simulink model "powerline_cycle_waterfall_milestone_06"  (R2026a)
settings: Solver=VariableStepAuto  StopTime=59/60
model workspace (MAT data in the model file):
  noiseGain = 1
  sparkGain = 1
undefined symbols (not defined in the file): fs
libraries: dspsrcs4 x3
settings Model: PacingRate=0.100000  Creator=docto  LastModifiedBy=docto

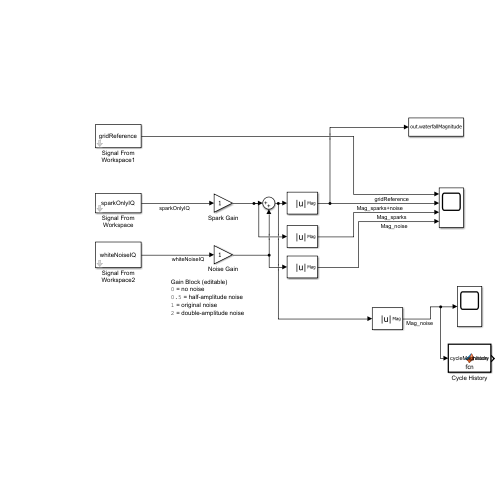
[thumbnail: Simulink's stored preview of the top-level diagram]
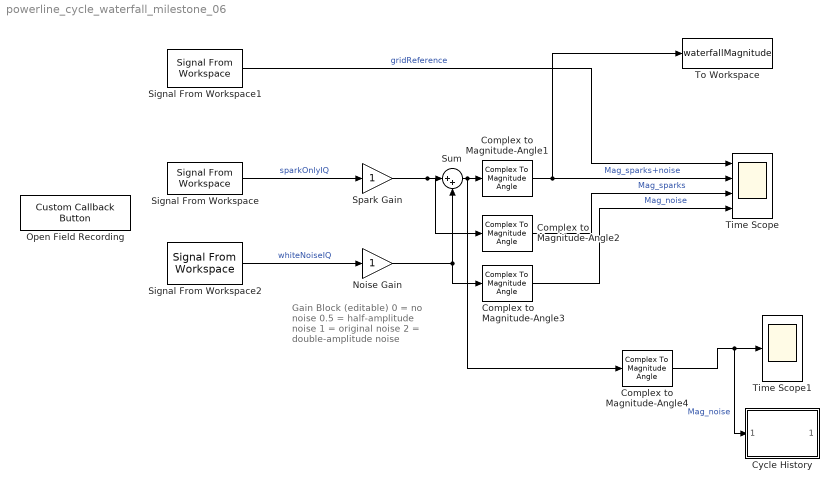
== system powerline_cycle_waterfall_milestone_06 ==
  note: Gain Block (editable)
      | 0 = no noise
      | 0.5 = half-amplitude noise
      | 1 = original noise
      | 2 = double-amplitude noise
  Complex to Magnitude-Angle{1..4} (4 alike) : ComplexToMagnitudeAngle  Output=Magnitude
  Cycle History : MATLAB Function  TreatAsAtomicUnit=on
  Noise Gain : Gain
  Open Field Recording : CustomCallbackButton  Configuration="{\"components\":[{\"name\":\"BackgroundImageComponent\",\"settings\":{\"image\":{\"size\":[0,0],\"src\":\"default\",\"srcOrientation\":\"Right\"},\"position\":[0,0,1,1]}},{\"name\":\"ButtonStateComponent\",\"settings\":{\"buttonType\":\"momentary\",\"clickFcn\":\"openFieldEventWaterfall;\",\"onValue\":1,\"position\":[0,0,1,1],\"pressDelay\":\"500\",\"pressFcn\":\"\",\"repeatInterval\":\"0\",\"states\":[{\"horizontalAlignment\":\"center\",\"image\":{\"position\":[0,0,1,1],\"size\":[1,1],\"src\":\"default\",\"srcOrientation\":\"Right\"},\"label\":{\"color\":[0.01176470588,0.01176470588,0.01176470588,1],\"icon\":{\"size\":[0,0],\"src\":\"default\",\"srcOrientation\":\"Right\"},\"iconOffset\":0,\"iconPlacement\":\"left\",\"opacity\":1,\"show\":true,\"text\":{\"content\":\"Open Field Recording\",\"font\":\"Helvetica\"}},\"labelOffset\":[0,0],\"verticalAlignment\":\"middle\"},{\"horizontalAlignment\":\"center\",\"image\":{\"position\":[0,0,1,1],\"size\":[1,1],\"src\":\"default\",\"srcOrientation\":\"Right\"},\"label\":{\"color\":[0.01176470588,0.01176470588,0.01176470588,1],\"icon\":{\"size\":[0,0],\"src\":\"default\",\"srcOrientation\":\"Right\"},\"iconOffset\":0,\"iconPlacement\":\"left\",\"opacity\":1,\"show\":true,\"text\":{\"content\":\"Open Field Recording\",\"font\":\"Helvetica\"}},\"labelOffset\":[0,0],\"verticalAlignment\":\"middle\"},{\"horizontalAlignment\":\"center\",\"image\":{\"position\":[0,0,1,1],\"size\":[1,1],\"src\":\"default\",\"srcOrientation\":\"Right\"},\"label\":{\"color\":[0.01176470588,0.01176470588,0.01176470588,1],\"icon\":{\"size\":[0,0],\"src\":\"default\",\"srcOrientation\":\"Right\"},\"iconOffset\":0,\"iconPlacement\":\"left\",\"opacity\":1,\"show\":true,\"text\":{\"content\":\"Open Field Recording\",\"font\":\"Helvetica\"}},\"labelOffset\":[0,0],\"verticalAlignment\":\"middle\"},{\"horizontalAlignment\":\"center\",\"image\":{\"position\":[0,0,1,1],\"size\":[1,1],\"src\":\"default\",\"srcOrientation\":\"Right\"},\"label\":{\"color\":[0.01176470588,0.01176470588,0.01176470588,1],\"icon\":{\"size\":[0,0],\"src\":\"default\",\"srcOrientation\":\"Right\"},\"iconOffset\":0,\"iconPlacement\":\"left\",\"opacity\":1,\"show\":true,\"text\":{\"content\":\"Open Field Recording\",\"font\":\"Helvetica\"}},\"labelOffset\":[0,0],\"verticalAlignment\":\"middle\"}]}},{\"name\":\"ForegroundImageComponent\",\"settings\":{\"image\":{\"size\":[0,0],\"src\":\"default\",\"srcOrientation\":\"Right\"},\"isForeground\":1,\"position\":[0,0,1,1]}}],\"derived\":{\"blockParameters\":{\"AutoActivate\":true,\"ButtonText\":\"Open Field Recording\",\"ButtonType\":\"Momentary\",\"ClickFcn\":\"openFieldEventWaterfall;\",\"OnValue\":1,\"PressDelay\":\"500\",\"PressFcn\":\"\",\"RepeatInterval\":\"0\",\"fixedAspectRatio\":\"off\"}},\"settings\":{\"BindingType\":\"standalone\",\"autoActivate\":true,\"backgroundColor\":[244,244,244,1],\"backgroundOffset\":0.2,\"backgroundOpacity\":1,\"fixedAspectRatio\":\"off\",\"foregroundColor\":[0.01176470588,0.01176470588,0.01176470588,1],\"migratedFromLegacy\":true,\"useBackgroundColor\":true,\"variant\":\"callback\",\"version\":\"R2025a\"},\"type\":\"Button\"}"  CustomBackgroundColor="{\"color\":[0.9568627451,0.9568627451,0.9568627451],\"show\":true}"
  Signal From Workspace : dspsrcs4/Signal From Workspace  X=sparkOnlyIQ  Ts=1/fs  nsamps=40000  OutputAfterFinalValue=Setting to zero  ignoreOrWarnInputAndFrameLengths=off  OutputFrames=off
  Signal From Workspace1 : dspsrcs4/Signal From Workspace  X=gridReference  Ts=1/fs  nsamps=40000  OutputAfterFinalValue=Setting to zero  ignoreOrWarnInputAndFrameLengths=off  OutputFrames=off
  Signal From Workspace2 : dspsrcs4/Signal From Workspace  X=whiteNoiseIQ  Ts=1/fs  nsamps=40000  OutputAfterFinalValue=Setting to zero  ignoreOrWarnInputAndFrameLengths=off  OutputFrames=off
  Spark Gain : Gain
  Sum : Sum  Inputs=|++
  Time Scope : Scope  NumInputPorts=4
      settings: TimeSpan=One frame period  TimeUnits=Metric (based on Time Span)  ActiveDisplayString=4  ActiveDisplayYMinimum=-0.0089837498962879164  ActiveDisplayYMaximum=0.080853749066591263  YLabel=Amplitude
  Time Scope1 : Scope
      settings: TimeSpan=One frame period  TimeUnits=Metric (based on Time Span)  ActiveDisplayYMinimum=0  ActiveDisplayYMaximum=0.35  YLabel=Amplitude
  To Workspace : ToWorkspace  VariableName=waterfallMagnitude  SaveFormat=Timeseries  SampleTime=-1
  wires:
  Signal From Workspace1/1 -> Time Scope/1  "gridReference"
  Spark Gain/1 -> Complex to Magnitude-Angle2/1, Sum/1
  Noise Gain/1 -> Complex to Magnitude-Angle3/1, Sum/2
  Complex to Magnitude-Angle1/1 -> To Workspace/1, Time Scope/2  "Mag_sparks+noise"
  Signal From Workspace/1 -> Spark Gain/1  "sparkOnlyIQ"
  Signal From Workspace2/1 -> Noise Gain/1  "whiteNoiseIQ"
  Complex to Magnitude-Angle3/1 -> Time Scope/4  "Mag_noise"
  Complex to Magnitude-Angle2/1 -> Time Scope/3  "Mag_sparks"
  Sum/1 -> Complex to Magnitude-Angle4/1, Complex to Magnitude-Angle1/1
  Complex to Magnitude-Angle4/1 -> Cycle History/1(cycleMagnitude), Time Scope1/1  "Mag_noise"

== matlab function powerline_cycle_waterfall_milestone_06/Cycle History ==
  data: cycleMagnitude input; history output
function history = fcn(cycleMagnitude)
%#codegen

persistent H
row = zeros(1,2000,'single');

if isempty(H)
    H = zeros(60,2000,'single');
end

for k = 1:2000
    first = (k-1)*20 + 1;
    row(k) = max(single(cycleMagnitude(first:first+19)));
end

H(1:59,:) = H(2:60,:);
H(60,:) = row;

history = H;
